simulink model "gim_ut"  (Simulink 8.1)
settings: Solver=FixedStepDiscrete  StartTime=0.0  StopTime=10.0  FixedStep=0.005  RelTol=1e-3
libraries: siltestlib x29, idiada_lib x5, gim x1
settings Model: Creator=xsellart  LastModifiedBy=AT015555
settings DataIOCC: SignalLoggingSaveFormat=Dataset
settings OptimizationCC: ExpressionDepthLimit=128
settings DebuggingCC: FcnCallInpInsideContextMsg=EnableAllAsError
settings GRTTargetCC: CombineOutputUpdateFcns=on  GRTInterface=off

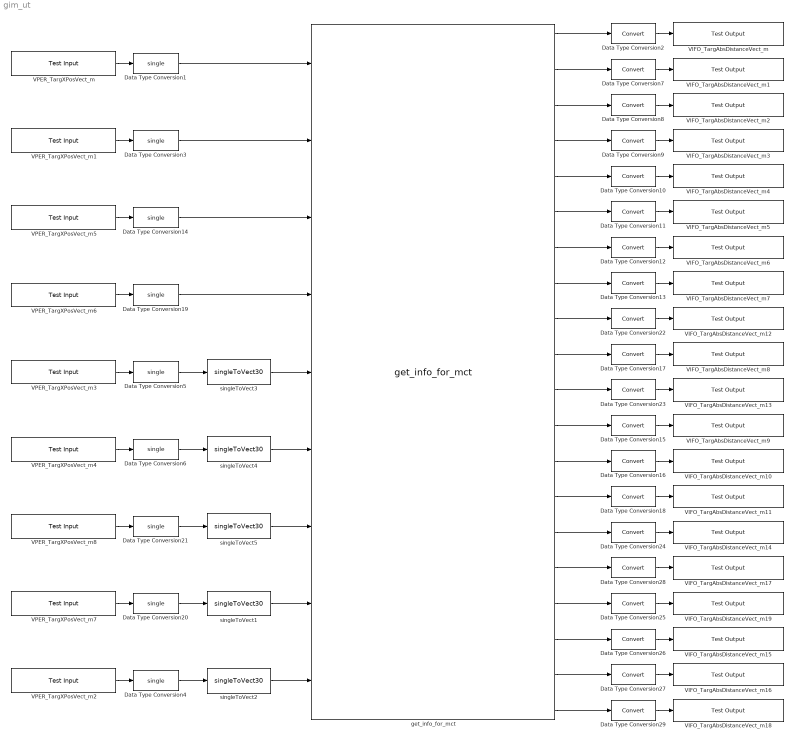
== system gim_ut ==
  Data Type Conversion{1,3..6,14,19..21} (9 alike) : DataTypeConversion  OutDataTypeStr=single
  Data Type Conversion{2,7..13,15..18,22..29} (20 alike) : DataTypeConversion
  VIFO_TargAbsDistanceVect_m : siltestlib/Test Output  varname=VIFO_FCWTargetVehRelSpeedX_mps  sampletime=-1
  VIFO_TargAbsDistanceVect_m1 : siltestlib/Test Output  varname=VIFO_FCWMCVehXPosition_m  sampletime=-1
  VIFO_TargAbsDistanceVect_m10 : siltestlib/Test Output  varname=VIFO_ACCTargetVehAssigned_flg  sampletime=-1
  VIFO_TargAbsDistanceVect_m11 : siltestlib/Test Output  varname=VIFO_ACCMCVehId_num  sampletime=-1
  VIFO_TargAbsDistanceVect_m12 : siltestlib/Test Output  varname=VIFO_FCWMCLongAccel_mps2  sampletime=-1
  VIFO_TargAbsDistanceVect_m13 : siltestlib/Test Output  varname=VIFO_ACCTargetVehRelSpeedX_mps  sampletime=-1
  VIFO_TargAbsDistanceVect_m14 : siltestlib/Test Output  varname=VIFO_ACCMCLongAccel_mps2  sampletime=-1
  VIFO_TargAbsDistanceVect_m15 : siltestlib/Test Output  varname=VIFO_VRUTargetPedAssigned_flg  sampletime=-1
  VIFO_TargAbsDistanceVect_m16 : siltestlib/Test Output  varname=VIFO_VRUMCPedId_num  sampletime=-1
  VIFO_TargAbsDistanceVect_m17 : siltestlib/Test Output  varname=VIFO_VRUTargetPedRelSpeedX_mps  sampletime=-1
  VIFO_TargAbsDistanceVect_m18 : siltestlib/Test Output  varname=VIFO_VRUMCLongAccel_mps2  sampletime=-1
  VIFO_TargAbsDistanceVect_m19 : siltestlib/Test Output  varname=VIFO_VRUMCPedXPosition_m  sampletime=-1
  VIFO_TargAbsDistanceVect_m2 : siltestlib/Test Output  varname=VIFO_FCWTargetVehAssigned_flg  sampletime=-1
  VIFO_TargAbsDistanceVect_m3 : siltestlib/Test Output  varname=VIFO_AEBTargetVehRelSpeedX_mps  sampletime=-1
  VIFO_TargAbsDistanceVect_m4 : siltestlib/Test Output  varname=VIFO_AEBMCVehXPosition_m  sampletime=-1
  VIFO_TargAbsDistanceVect_m5 : siltestlib/Test Output  varname=VIFO_AEBTargetVehAssigned_flg  sampletime=-1
  VIFO_TargAbsDistanceVect_m6 : siltestlib/Test Output  varname=VIFO_FCWMCVehId_num  sampletime=-1
  VIFO_TargAbsDistanceVect_m7 : siltestlib/Test Output  varname=VIFO_AEBMCVehId_num  sampletime=-1
  VIFO_TargAbsDistanceVect_m8 : siltestlib/Test Output  varname=VIFO_AEBMCLongAccel_mps2  sampletime=-1
  VIFO_TargAbsDistanceVect_m9 : siltestlib/Test Output  varname=VIFO_ACCMCVehXPosition_m  sampletime=-1
  VPER_TargXPosVect_m : siltestlib/Test Input  varname=VIFO_FCWMCTTargetId_enum  sampletime=0.005
  VPER_TargXPosVect_m1 : siltestlib/Test Input  varname=VIFO_AEBMCTTargetId_enum  sampletime=0.005
  VPER_TargXPosVect_m2 : siltestlib/Test Input  varname=VPER_TargXPosVect30_m  sampletime=0.005
  VPER_TargXPosVect_m3 : siltestlib/Test Input  varname=VIFO_TargVehRelSpdXVect30_mps  sampletime=0.005
  VPER_TargXPosVect_m4 : siltestlib/Test Input  varname=VPER_TargIdVect30_num  sampletime=0.005
  VPER_TargXPosVect_m5 : siltestlib/Test Input  varname=VIFO_ACCMCTTargetId_enum  sampletime=0.005
  VPER_TargXPosVect_m6 : siltestlib/Test Input  varname=VIFO_VRUMCTTargetId_enum  sampletime=0.005
  VPER_TargXPosVect_m7 : siltestlib/Test Input  varname=VPER_TargXPosVect30_m  sampletime=0.005
  VPER_TargXPosVect_m8 : siltestlib/Test Input  varname=VIFO_TargAccelXVect30_mps2  sampletime=0.005
  get_info_for_mct : gim/get_info_for_mct
  singleToVect{1..5} (5 alike) : idiada_lib/singleToVect30
  wires:
  VPER_TargXPosVect_m/1 -> Data Type Conversion1/1
  Data Type Conversion1/1 -> get_info_for_mct/1
  get_info_for_mct/1 -> Data Type Conversion2/1
  Data Type Conversion2/1 -> VIFO_TargAbsDistanceVect_m/1
  VPER_TargXPosVect_m1/1 -> Data Type Conversion3/1
  Data Type Conversion3/1 -> get_info_for_mct/2
  VPER_TargXPosVect_m2/1 -> Data Type Conversion4/1
  Data Type Conversion4/1 -> singleToVect2/1
  VPER_TargXPosVect_m3/1 -> Data Type Conversion5/1
  Data Type Conversion5/1 -> singleToVect3/1
  VPER_TargXPosVect_m4/1 -> Data Type Conversion6/1
  Data Type Conversion6/1 -> singleToVect4/1
  get_info_for_mct/2 -> Data Type Conversion7/1
  Data Type Conversion7/1 -> VIFO_TargAbsDistanceVect_m1/1
  get_info_for_mct/3 -> Data Type Conversion8/1
  Data Type Conversion8/1 -> VIFO_TargAbsDistanceVect_m2/1
  get_info_for_mct/4 -> Data Type Conversion9/1
  Data Type Conversion9/1 -> VIFO_TargAbsDistanceVect_m3/1
  get_info_for_mct/5 -> Data Type Conversion10/1
  Data Type Conversion10/1 -> VIFO_TargAbsDistanceVect_m4/1
  Data Type Conversion11/1 -> VIFO_TargAbsDistanceVect_m5/1
  Data Type Conversion12/1 -> VIFO_TargAbsDistanceVect_m6/1
  Data Type Conversion13/1 -> VIFO_TargAbsDistanceVect_m7/1
  singleToVect2/1 -> get_info_for_mct/9
  singleToVect3/1 -> get_info_for_mct/5
  singleToVect4/1 -> get_info_for_mct/6
  VPER_TargXPosVect_m5/1 -> Data Type Conversion14/1
  Data Type Conversion14/1 -> get_info_for_mct/3
  Data Type Conversion17/1 -> VIFO_TargAbsDistanceVect_m8/1
  Data Type Conversion15/1 -> VIFO_TargAbsDistanceVect_m9/1
  Data Type Conversion16/1 -> VIFO_TargAbsDistanceVect_m10/1
  Data Type Conversion18/1 -> VIFO_TargAbsDistanceVect_m11/1
  VPER_TargXPosVect_m6/1 -> Data Type Conversion19/1
  Data Type Conversion19/1 -> get_info_for_mct/4
  VPER_TargXPosVect_m7/1 -> Data Type Conversion20/1
  Data Type Conversion20/1 -> singleToVect1/1
  VPER_TargXPosVect_m8/1 -> Data Type Conversion21/1
  Data Type Conversion21/1 -> singleToVect5/1
  singleToVect5/1 -> get_info_for_mct/7
  singleToVect1/1 -> get_info_for_mct/8
  Data Type Conversion22/1 -> VIFO_TargAbsDistanceVect_m12/1
  get_info_for_mct/6 -> Data Type Conversion11/1
  get_info_for_mct/7 -> Data Type Conversion12/1
  get_info_for_mct/8 -> Data Type Conversion13/1
  get_info_for_mct/9 -> Data Type Conversion22/1
  get_info_for_mct/10 -> Data Type Conversion17/1
  get_info_for_mct/11 -> Data Type Conversion23/1
  Data Type Conversion23/1 -> VIFO_TargAbsDistanceVect_m13/1
  get_info_for_mct/12 -> Data Type Conversion15/1
  get_info_for_mct/13 -> Data Type Conversion16/1
  get_info_for_mct/14 -> Data Type Conversion18/1
  Data Type Conversion24/1 -> VIFO_TargAbsDistanceVect_m14/1
  get_info_for_mct/15 -> Data Type Conversion24/1
  Data Type Conversion25/1 -> VIFO_TargAbsDistanceVect_m19/1
  Data Type Conversion26/1 -> VIFO_TargAbsDistanceVect_m15/1
  Data Type Conversion27/1 -> VIFO_TargAbsDistanceVect_m16/1
  Data Type Conversion28/1 -> VIFO_TargAbsDistanceVect_m17/1
  Data Type Conversion29/1 -> VIFO_TargAbsDistanceVect_m18/1
  get_info_for_mct/16 -> Data Type Conversion28/1
  get_info_for_mct/17 -> Data Type Conversion25/1
  get_info_for_mct/18 -> Data Type Conversion26/1
  get_info_for_mct/19 -> Data Type Conversion27/1
  get_info_for_mct/20 -> Data Type Conversion29/1
